simulink model "pro4"  (R2020b)
settings: Solver=VariableStepAuto  StartTime=0.0  StopTime=10.0  RelTol=1e-3
model workspace (MAT data in the model file):
  a = Simulink.Parameter
  a.Value = 1
  a.DataType = 'auto'
  a.Dimensions = [1 1]
  b = Simulink.Parameter
  b.Value = 1
  b.DataType = 'auto'
  b.Dimensions = [1 1]
  c = Simulink.Parameter
  c.Value = 0.5
  c.DataType = 'auto'
  c.Dimensions = [1 1]
  d = Simulink.Parameter
  d.Value = 0.4
  d.DataType = 'auto'
  d.Dimensions = [1 1]
  e = Simulink.Parameter
  e.Value = -0.25
  e.DataType = 'auto'
  e.Dimensions = [1 1]
settings Model: Creator=sushma  LastModifiedBy=sushma

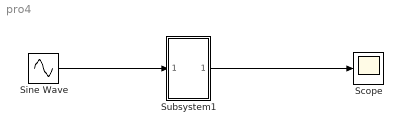
== system pro4 ==
  Scope : Scope
  Sine Wave : Sin  SampleTime=0
  Subsystem1 : ModelReference  ModelNameDialog=Subsystem10  SimulationMode=Normal  ModelReferenceVersion=1.3
  wires:
  Sine Wave/1 -> Subsystem1/1
  Subsystem1/1 -> Scope/1
